simulink model "Planar_2R"  (R2018a)
settings: Solver=VariableStepAuto  StartTime=0.0  StopTime=22  FixedStep=1/1000  RelTol=1e-6
values from neighbouring files (symbols this model uses):
  A = double(vpa(A, 5))    [planar_2r.m]
  B = double(vpa(B, 5))    [planar_2r.m]
  C = [1 0 0 0; 0 0 1 0]    [planar_2r.m]
  D = zeros(size(C,1), size(C,1))    [planar_2r.m]
  K = [Kt(1, 1:size(A,1)); Kt(2, 1:size(A,1))]    [planar_2r.m]
  Ka = [-Kt(1,end-(size(B,2)-1):end); -Kt(2, end-(size(B,2)-1):end)]    [planar_2r.m]
  L = [1 0; 0 1; 1 0; 0 1]    [planar_2r.m]
  Tau_op = double(Tau_op)'    [planar_2r.m]
  Tobs = lyap(-Fobs, A, -L*C)    [planar_2r.m]
undefined symbols (not defined in the file or in its folder): Fobs, X_op
libraries: simulink x2
settings Model: Creator=Mauricio  LastModifiedBy=Mauricio

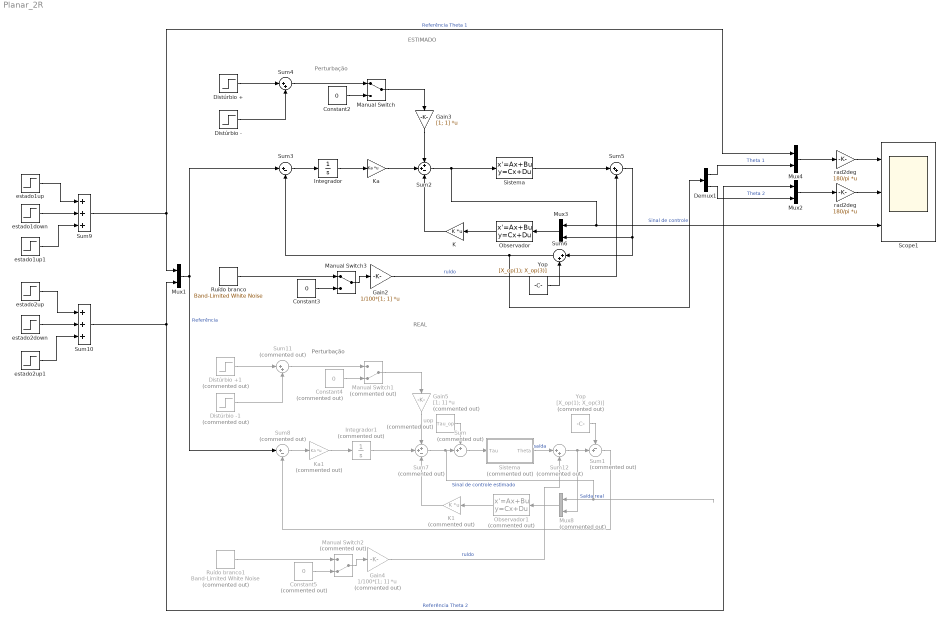
== system Planar_2R ==
  note: Perturbação
  note: ESTIMADO
  note: REAL
  note: Perturbação
  Constant2 : Constant  Value=0
  Constant3 : Constant  Value=0
  Constant4 : Constant  Commented=on  Value=0
  Constant5 : Constant  Commented=on  Value=0
  Demux1 : Demux  Outputs=[1 1]
  Distúrbio + : Step  Time=12  After=200  SampleTime=0.001
  Distúrbio +1 : Step  Commented=on  Time=3  After=200  SampleTime=0.001
  Distúrbio - : Step  Time=18  After=-200  SampleTime=0.001
  Distúrbio -1 : Step  Commented=on  Time=6  After=-200  SampleTime=0.001
  Gain2 : Gain  Gain=1/100*[1; 1]  Multiplication=Matrix(K*u)
  Gain3 : Gain  Gain=[1; 1]  Multiplication=Matrix(K*u)
  Gain4 : Gain  Commented=on  Gain=1/100*[1; 1]  Multiplication=Matrix(K*u)
  Gain5 : Gain  Commented=on  Gain=[1; 1]  Multiplication=Matrix(K*u)
  Integrador : Integrator
  Integrador1 : Integrator  Commented=on
  K : Gain  Gain=K  Multiplication=Matrix(K*u)
  K1 : Gain  Commented=on  Gain=K  Multiplication=Matrix(K*u)
  Ka : Gain  Gain=Ka  Multiplication=Matrix(K*u)
  Ka1 : Gain  Commented=on  Gain=Ka  Multiplication=Matrix(K*u)
  Manual Switch : ManualSwitch
  Manual Switch1 : ManualSwitch  Commented=on  CurrentSetting=0
  Manual Switch2 : ManualSwitch  Commented=on  CurrentSetting=0
  Manual Switch3 : ManualSwitch
  Mux{1..4} (4 alike) : Mux  Inputs=2
  Mux8 : Mux  Commented=on  Inputs=2
  Observador : StateSpace  A=Fobs  B=[Tobs*B L]  C=[inv(Tobs)]  D=zeros(size([Tobs*B L]))  InitialCondition=0
  Observador1 : StateSpace  Commented=on  A=Fobs  B=[Tobs*B L]  C=[inv(Tobs)]  D=zeros(size([Tobs*B L]))  InitialCondition=0
  Ruído branco : simulink/Sources/Band-Limited White Noise  Cov=[0.1]  Ts=0.01  seed=[23341]
  Ruído branco1 : simulink/Sources/Band-Limited White Noise  Commented=on  Cov=[0.1]  Ts=0.01  seed=[23341]
  Scope1 : Scope  NumInputPorts=3
  Sistema : StateSpace  A=A  B=B  C=C  D=D  InitialCondition=0
  "Sistema " : Subsystem  Commented=on
  Sum : Sum  Commented=on  Inputs=++|
  Sum1 : Sum  Commented=on  Inputs=-+|
  Sum10 : Sum  Inputs=+++
  Sum11 : Sum  Commented=on  Inputs=|++
  Sum12 : Sum  Commented=on  Inputs=|++
  Sum2 : Sum  Inputs=++-
  Sum3 : Sum  Inputs=|+-
  Sum4 : Sum  Inputs=|++
  Sum5 : Sum  Inputs=|++
  Sum6 : Sum  Inputs=|++
  Sum7 : Sum  Commented=on  Inputs=++-
  Sum8 : Sum  Commented=on  Inputs=|+-
  Sum9 : Sum  Inputs=+++
  Yop : Constant  Value=[X_op(1); X_op(3)]
  "Yop " : Constant  Commented=on  Value=[X_op(1); X_op(3)]
  estado1down : Step  Time=15  After=-X_op(1)*0.2
  estado1up : Step  Before=X_op(1)  After=X_op(1)*1.1
  estado1up1 : Step  Time=9  After=X_op(1)*0.1
  estado2down : Step  Time=15  After=-X_op(3)*0.2
  estado2up : Step  Time=5  Before=X_op(3)  After=X_op(3)*1.1
  estado2up1 : Step  Time=9  After=X_op(3)*0.1
  rad2deg : Gain  Gain=180/pi  Multiplication=Matrix(K*u)
  "rad2deg " : Gain  Gain=180/pi  Multiplication=Matrix(K*u)
  uop : Constant  Commented=on  Value=Tau_op
  wires:
  Sum4/1 -> Manual Switch/1
  K/1 -> Sum2/3
  Manual Switch/1 -> Gain3/1
  Integrador/1 -> Ka/1
  Mux1/1 -> Sum3/1, Sum8/1  "Referência"
  rad2deg/1 -> Scope1/1
  Sum2/1 -> Sistema/1, Scope1/3, Mux3/1  "Sinal de controle"
  Distúrbio -/1 -> Sum4/2
  Sum3/1 -> Integrador/1
  Distúrbio +/1 -> Sum4/1
  Ka/1 -> Sum2/2
  Ruído branco/1 -> Manual Switch3/1
  Constant2/1 -> Manual Switch/2
  Manual Switch3/1 -> Gain2/1
  Sistema/1 -> Sum5/1
  Observador/1 -> K/1
  Constant3/1 -> Manual Switch3/2
  Sum5/1 -> Mux3/2, Sum6/1
  Mux3/1 -> Observador/1
  Mux8/1 -> Observador1/1
  Distúrbio -1/1 -> Sum11/2
  Constant4/1 -> Manual Switch1/2
  Observador1/1 -> K1/1
  Manual Switch2/1 -> Gain4/1
  Sum8/1 -> Ka1/1
  Distúrbio +1/1 -> Sum11/1
  Constant5/1 -> Manual Switch2/2
  Gain5/1 -> Sum7/1
  K1/1 -> Sum7/3
  Ruído branco1/1 -> Manual Switch2/1
  Sum11/1 -> Manual Switch1/1
  Sum7/1 -> Mux8/1, Sum/2  "Sinal de controle estimado"
  Manual Switch1/1 -> Gain5/1
  "Yop "/1 -> Sum1/1
  Ka1/1 -> Integrador1/1
  Integrador1/1 -> Sum7/2
  Sum12/1 -> Mux8/2, Sum1/2  "Saída real"
  Sum6/1 -> Demux1/1, Sum3/2
  Yop/1 -> Sum6/2
  "Sistema "/1(Theta) -> Sum12/1  "saída"
  Sum/1 -> "Sistema "/1(Tau)
  uop/1 -> Sum/1
  Mux4/1 -> rad2deg/1
  Sum1/1 -> Sum8/2
  Gain4/1 -> Sum12/2  "ruído"
  Gain2/1 -> Sum5/2  "ruído"
  Gain3/1 -> Sum2/1
  Sum9/1 -> Mux4/1, Mux1/1  "Referência Theta 1"
  estado1up/1 -> Sum9/1
  estado1down/1 -> Sum9/2
  Sum10/1 -> Mux1/2, Mux2/1  "Referência Theta 2"
  estado2up/1 -> Sum10/1
  estado2down/1 -> Sum10/2
  estado2up1/1 -> Sum10/3
  estado1up1/1 -> Sum9/3
  Demux1/1 -> Mux4/2  "Theta 1"
  Demux1/2 -> Mux2/2  "Theta 2"
  Mux2/1 -> "rad2deg "/1
  "rad2deg "/1 -> Scope1/2

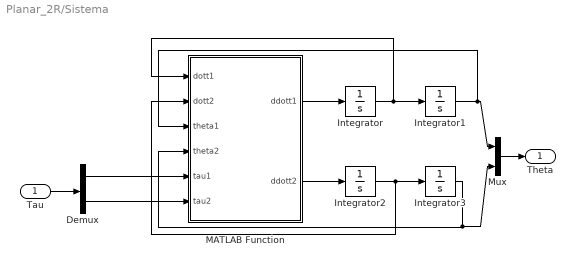
== system Planar_2R/Sistema  ==
  Tau : Inport
  Demux : Demux  Outputs=2
  Integrator : Integrator  InitialCondition=X_op(2)
  Integrator1 : Integrator  InitialCondition=X_op(1)
  Integrator2 : Integrator  InitialCondition=X_op(4)
  Integrator3 : Integrator  InitialCondition=X_op(3)
  MATLAB Function : MATLAB Function  TreatAsAtomicUnit=on
  Mux : Mux  Inputs=2
  Theta : Outport
  wires:
  MATLAB Function/2(ddott2) -> Integrator2/1
  Integrator/1 -> MATLAB Function/1(dott1), Integrator1/1
  Integrator2/1 -> MATLAB Function/2(dott2), Integrator3/1
  MATLAB Function/1(ddott1) -> Integrator/1
  Integrator1/1 -> Mux/1, MATLAB Function/3(theta1)
  Integrator3/1 -> MATLAB Function/4(theta2), Mux/2
  Mux/1 -> Theta/1
  Demux/2 -> MATLAB Function/6(tau2)
  Demux/1 -> MATLAB Function/5(tau1)
  Tau/1 -> Demux/1

== matlab function Planar_2R/Sistema /MATLAB Function ==
  data: dott1 input size=1; ddott1 output size=1; dott2 input size=1; theta1 input size=1; theta2 input size=1; tau1 input size=1; tau2 input size=1; ddott2 output size=1
function [ddott1,ddott2] = fcn(dott1,dott2,theta1,theta2,tau1,tau2)
m1 = 1;
m2 = 1;
l1 = 1;
l2 = 1;
g = 9.81;

f1 = ((sin(theta1)*cos(theta2) - cos(theta1)*sin(theta2))*(m2*l1*l2*(sin(theta1)*sin(theta2)+cos(theta1)*cos(theta2))*(dott1^2)-m2*(l2^2)*(dott2^2)))/(l1*l2*((m1+m2)-m2*(sin(theta1)*sin(theta2)+cos(theta1)*cos(theta2))^2)) + ((m1+m2)*l2*g*sin(theta1)-m2*l2*g*sin(theta2)*(sin(theta1)*sin(theta2)+cos(theta1)*cos(theta2)))/(l1*l2*((m1+m2)-m2*(sin(theta1)*sin(theta2)+cos(theta1)*cos(theta2))^2));
f2 = ((sin(theta1)*cos(theta2) - cos(theta1)*sin(theta2))*(-(m1+m2)*(l1^2)*(dott1^2)+m2*l1*l2*(sin(theta1)*sin(theta2)+cos(theta1)*cos(theta2))*(dott2^2)))/(l1*l2*((m1+m2)-m2*(sin(theta1)*sin(theta2)+cos(theta1)*cos(theta2))^2)) + (-(m1+m2)*l1*g*sin(theta1)*(sin(theta1)*sin(theta2)+cos(theta1)*cos(theta2))+(m1+m2)*l1*g*sin(theta2))/(l1*l2*((m1+m2)-m2*(sin(theta1)*sin(theta2)+cos(theta1)*cos(theta2))^2));

g11 = (m2*l2^2)/(m2*(l1^2)*(l2^2)*((m1+m2)-m2*(sin(theta1)*sin(theta2)+cos(theta1)*cos(theta2))^2));
g12 = (-m2*l1*l2*(sin(theta1)*sin(theta2)+cos(theta1)*cos(theta2)))/(m2*(l1^2)*(l2^2)*((m1+m2)-m2*(sin(theta1)*sin(theta2)+cos(theta1)*cos(theta2))^2));
g21 = g12;
g22 = ((m1+m2)*(l1^2))/(m2*(l1^2)*(l2^2)*((m1+m2)-m2*(sin(theta1)*sin(theta2)+cos(theta1)*cos(theta2))^2));

% f1 = (sin(theta1)*cos(theta2) - cos(theta1)*sin(theta2))/(l1*l2*((m1+m2)-m2*(sin(theta1)*sin(theta2)+cos(theta1)*cos(theta2))^2)*(m2*l1*l2*(sin(theta1)*sin(theta2)+cos(theta1)*cos(theta2))*(dott1^2)-m2*(l2^2)*(dott2^2))) + 1/(l1*l2*((m1+m2)-m2*(sin(theta1)*sin(theta2)+cos(theta1)*cos(theta2))^2)*((m1+m2)*l2*g*sin(theta1)-m2*l2*g*sin(theta2)*(sin(theta1)*sin(theta2)+cos(theta1)*cos(theta2))));
% f2 = (sin(theta1)*cos(theta2) - cos(theta1)*sin(theta2))/(l1*l2*((m1+m2)-m2*(sin(theta1)*sin(theta2)+cos(theta1)*cos(theta2))^2)*(-(m1+m2)*(l1^2)*(dott1^2)+m2*l1*l2*(sin(theta1)*sin(theta2)+cos(theta1)*cos(theta2))*(dott2^2))) + 1/(l1*l2*((m1+m2)-m2*(sin(theta1)*sin(theta2)+cos(theta1)*cos(theta2))^2)*(-(m1+m2)*l1*g*sin(theta1)*(sin(theta1)*sin(theta2)+cos(theta1)*cos(theta2))+(m1+m2)*l1*g*sen(theta2)));
% 
% g11 = (m2*l2^2)/(m2*(l1^2)*(l2^2)*((m1+m2)-m2*(sin(theta1)*sin(theta2)+cos(theta1)*cos(theta2))^2));
% g12 = (-m2*l1*l2*(sin(theta1)*sin(theta2)+cos(theta1)*cos(theta2)))/(m2*(l1^2)*(l2^2)*((m1+m2)-m2*(sin(theta1)*sin(theta2)+cos(theta1)*cos(theta2))^2));
% g21 = g12;
% g22 = ((m1+m2)*(l1^2))/(m2*(l1^2)*(l2^2)*((m1+m2)-m2*(sin(theta1)*sin(theta2)+cos(theta1)*cos(theta2))^2));

ddott1 = f1 + g11*tau1 + g12*tau2;
ddott2 = f2 + g21*tau1 + g22*tau1;
